simulink model "Quaternions_Method_merge_gio_giusto"  (R2021b)
settings: Solver=FixedStepAuto  StartTime=0.0  StopTime=Time  FixedStep=1  RelTol=1e-13  AbsTol=1e-8
values from neighbouring files (symbols this model uses):
  a = 8.6251e+06    (= 8625100)    [Main.m]
  c = 299792*10^3    (= 299792000)    [Main.m]
  e = 0.1195    [Main.m]
  G = 6.67259 * 1e-11    (= 6.67259e-11)    [Main.m]
  H_0 = sqrt((g_1_0)^2 + (g_1_1)^2 + (h_1_1)^2)    [Main.m]
  i = 0.3815    [Main.m]
  MB = [2000; 0.3; 1; 0.12].*1e-2    [Main.m]
  mr = 1.2 * 0.0001    (= 0.00012)    [Main.m]
  muP = G*Mt    (= 398527110340000)    [Main.m]
  omega_0 = [om_x, om_y, om_z]    [Main.m]
  p_acc = deg2rad(5)    [Main.m]
  RD = 0.1*ones(1,10)    [Main.m]
  RS_MB = 0.5    [Main.m]
  RS_SP = 0.1    [Main.m]
  SP = [2000; 0.3; 1; 0.12].*1e-2    [Main.m]
  theta0 = 0    [Main.m]
  w_E = (2*pi)/(24*3600)    (= 7.27220521664e-05)    [Main.m]
undefined symbols (not defined in the file or in its folder): A_BN_0, A_rw, A_rw_star, H, magnitude, rho_d_MB, rho_d_SP, rho_s_MB, rho_s_SP, sig_b, sig_n, T, t_sample
libraries: matrix_library x23, vrlib x9, simulink_extras x2, simulink x2
(part 8 of 8)

== system Quaternions_Method_merge_gio_giusto/Enviroment/Solar Radiation Perturbation/Sum forces/determine highlighted area/creazione della matrice che ha per colonne i vettori distanza tra il CM del MB e i centri geom delle aree illuminate dal sole /creazione raggi vettore tra CM MB e centro facce illuminate della faccia che ha come normale l'asse k/If Action Subsystem3 ==
  Action Port : ActionPort
  Constant : Constant  Value=[0;0;0]
  Out1 : Outport
  wires:
  Constant/1 -> Out1/1

== system Quaternions_Method_merge_gio_giusto/Enviroment/Solar Radiation Perturbation/Sum forces/determine highlighted area/creazione della matrice che ha per colonne i vettori distanza tra il CM del MB e i centri geom delle aree illuminate dal sole /creazione raggi vettore tra CM MB e centro facce illuminate della faccia che ha come normale l'asse k/If Action Subsystem4 ==
  Areas_vect : Inport
  MB1 : Inport  Port=2
  Action Port : ActionPort
  Add : Sum  Inputs=+|-
  Add1 : Sum  Inputs=+|-
  Add2 : Sum
  Demux : Demux  Outputs=3
  Demux1 : Demux  Outputs=3
  Demux2 : Demux
  Divide : Product  Inputs=*/
  Divide1 : Product  Inputs=*/
  Gain{,1..3} (4 alike) : Gain  Gain=1/2
  Gain4 : Gain  Gain=-1
  Ground : Ground
  Ground1 : Ground
  Mux : Mux  Inputs=3
  Mux1 : Mux  Inputs=3
  Reshape{,1..3} (4 alike) : Reshape  OutputDimensionality=Column vector (2-D)
  Terminator{,1..3,8..9} (6 alike) : Terminator
  r_cface_cluce_xneg_y_pos : Outport
  wires:
  Demux/2 -> Terminator8/1
  Demux/1 -> Terminator9/1
  Demux1/2 -> Terminator1/1
  Demux1/1 -> Terminator/1
  Add2/1 -> r_cface_cluce_xneg_y_pos/1
  Reshape3/1 -> Add2/2
  Reshape2/1 -> Add2/1
  Divide1/1 -> Gain3/1
  Reshape1/1 -> Demux1/1
  Gain2/1 -> Add1/1
  Gain3/1 -> Add1/2
  Demux1/3 -> Divide1/1
  Ground/1 -> Mux1/1, Mux1/3
  Mux1/1 -> Reshape3/1  "raggio vettore che collega il centro geom della faccia con il centro geom della faccia illuminata dal sole lungo j"
  Reshape/1 -> Demux/1
  Ground1/1 -> Mux/2, Mux/3
  Areas_vect/1 -> Reshape1/1, Reshape/1
  Gain/1 -> Add/1
  Demux/3 -> Divide/1
  Gain1/1 -> Add/2
  Mux/1 -> Reshape2/1  "raggio vettore che collega il centro geom della faccia con il centro geom della faccia illuminata dal sole lungo -i"
  Divide/1 -> Gain1/1
  [b_MB] -> Divide/2
  [a_MB] -> Gain/1
  Add/1 -> Gain4/1
  Gain4/1 -> Mux/1
  Add1/1 -> Mux1/2
  [b_MB] -> Gain2/1
  [a_MB] -> Divide1/2
  Demux2/1 -> Terminator2/1
  Demux2/2 -> [a_MB]
  MB1/1 -> Demux2/1
  Demux2/3 -> [b_MB]
  Demux2/4 -> Terminator3/1

== system Quaternions_Method_merge_gio_giusto/Enviroment/Solar Radiation Perturbation/Sum forces/determine highlighted area/creazione della matrice che ha per colonne i vettori distanza tra il CM del MB e i centri geom delle aree illuminate dal sole /creazione raggi vettore tra CM MB e centro facce illuminate della faccia che ha come normale l'asse k/If Action Subsystem5 ==
  Action Port : ActionPort
  Constant : Constant  Value=[0;0;0]
  Out1 : Outport
  wires:
  Constant/1 -> Out1/1

== system Quaternions_Method_merge_gio_giusto/Enviroment/Solar Radiation Perturbation/Sum forces/determine highlighted area/creazione della matrice che ha per colonne i vettori distanza tra il CM del MB e i centri geom delle aree illuminate dal sole /creazione raggi vettore tra CM MB e centro facce illuminate della faccia che ha come normale l'asse k/If Action Subsystem6 ==
  Action Port : ActionPort
  Constant : Constant  Value=[0;0;0]
  Out1 : Outport
  wires:
  Constant/1 -> Out1/1

== system Quaternions_Method_merge_gio_giusto/Enviroment/Solar Radiation Perturbation/Sum forces/determine highlighted area/creazione della matrice che ha per colonne i vettori distanza tra il CM del MB e i centri geom delle aree illuminate dal sole /creazione raggi vettore tra CM MB e centro facce illuminate della faccia che ha come normale l'asse k/If Action Subsystem7 ==
  Action Port : ActionPort
  Constant : Constant  Value=[0;0;0]
  Out1 : Outport
  wires:
  Constant/1 -> Out1/1

== system Quaternions_Method_merge_gio_giusto/Enviroment/Solar Radiation Perturbation/Sum forces/determine highlighted area/creazione della matrice che ha per colonne i vettori distanza tra il CM del MB e i centri geom delle aree illuminate dal sole /creazione raggi vettore tra CM MB e centro facce illuminate della faccia che ha come normale l'asse k/creating distance between cm MB and centro geom lato1 ==
  MB : Inport
  Demux : Demux
  Ground : Ground
  Mux : Mux  Inputs=3
  Reshape : Reshape  OutputDimensionality=Column vector (2-D)
  Terminator : Terminator
  Terminator2 : Terminator
  Terminator3 : Terminator
  Out1 : Outport
  wires:
  Reshape/1 -> Out1/1
  Mux/1 -> Reshape/1
  MB/1 -> Demux/1
  Demux/1 -> Terminator/1
  Demux/2 -> Mux/1
  Demux/3 -> Terminator2/1
  Ground/1 -> Mux/2, Mux/3
  Demux/4 -> Terminator3/1

== matlab function Quaternions_Method_merge_gio_giusto/Attitude determination/MATLAB Function ==
  data: K input; V output; D output
function [V, D] = fcn(K)
[V,D] = eig(K);
end

== matlab function Quaternions_Method_merge_gio_giusto/Enviroment/Magnetic torque /Magnetic field in body frame/MATLAB Function ==
  data: r_LVLH input; r input; b_N output; t input; G input; H input
function b_N  = magnet(r_LVLH, r, t, G, H)
% Inputs
% r Geocentric radius
% theta Latitude measured in degrees positive from equator
% phi Longitude measured in degrees positive east from Greenwich
%
% Outputs - magnetic field strength in local tangential coordinates
% Br B in radial direction
% Bt B in theta direction
% Bp B in phi direction

% Computing the right ascension alpha, the declination delta, the longitude lon and the co-latitude phi
r_norm = norm(r_LVLH);
delta = asin(r_LVLH(3)/r_norm);
if(r_LVLH(2)/r_norm > 0)
    alpha = acos((r_LVLH(1)/r_norm)/cos(delta));
else 
    alpha = 2*pi -  acos((r_LVLH(1)/r_norm)/cos(delta));
end
theta = -delta;
om_E = deg2rad(15.04)/3600;
Gren_lon = om_E*t;
phi = (alpha - Gren_lon);

% Checks to see if located at either pole to avoid singularities
if (theta>-0.00000001 && theta<0.00000001)
theta=0.00000001;
elseif(theta<180.00000001 && theta>179.99999999)
theta=179.99999999;
end
% The angles must be converted from degrees into radians
theta=(90-theta)*pi/180;
phi = phi*pi/180;
a=6371.2; % Reference radius used in IGRF
% This section of the code simply reads in the g and h Schmidt
% quasi-normalized coefficients
gn = G(:,1);
gm = G(:,2);
gvali = G(:,3);
hn = H(:,1);
hm = H(:,2);
hvali = H(:,3);
%[gn, gm, gvali, ~] = textread('igrfSg.txt','%f %f %f %f');
%[hn, hm, hvali, ~]= textread('igrfSh.txt','%f %f %f %f');
N=max(gn);
g=zeros(N,N+1);
h=zeros(N,N+1);
for x=1:length(gn)
g(gn(x),gm(x)+1) = gvali(x);
h(hn(x),hm(x)+1) = hvali(x);
end
% Initialize each of the variables
% Br B in the radial driection
% Bt B in the theta direction
% Bp B in the phi direction
% P The associated Legendre polynomial evaluated at cos(theta)
% The nomenclature for the recursive values generally follows
% the form P10 = P(n-1,m-0)
% dP The partial derivative of P with respect to theta
Br=0; Bt=0; Bp=0;
P11=1; P10=P11;
dP11=0; dP10=dP11;
for m=0:N
for n=1:N
if m<=n
% Calculate Legendre polynomials and derivatives recursively
if n==m
P2 = sin(theta)*P11;
dP2 = sin(theta)*dP11 + cos(theta)*P11;
P11=P2; P10=P11; P20=0;
dP11=dP2; dP10=dP11; dP20=0;
elseif n==1
P2 = cos(theta)*P10;
dP2 = cos(theta)*dP10 - sin(theta)*P10;
P20=P10; P10=P2;
dP20=dP10; dP10=dP2;
else
P20=P10;
dP20=dP10;
K = ((n-1)^2-m^2)/((2*n-1)*(2*n-3));
P2 = cos(theta)*P10 - K*P20;
dP2 = cos(theta)*dP10 - sin(theta)*P10 - K*dP20;
P10=P2;
dP10=dP2;
end
% Calculate Br, Bt, and Bp
Br = Br + (a/r)^(n+2)*(n+1)*...
((g(n,m+1)*cos(m*phi) + h(n,m+1)*sin(m*phi))*P2);
Bt = Bt + (a/r)^(n+2)*...
((g(n,m+1)*cos(m*phi) + h(n,m+1)*sin(m*phi))*dP2);
Bp = Bp + (a/r)^(n+2)*...
(m*(-g(n,m+1)*sin(m*phi) + h(n,m+1)*cos(m*phi))* P2);
end
end
end
% Spherical coordinates
Br = Br;
Bt = -Bt;
Bp = -Bp / sin(theta);

% Inertial cartesian coordinates
LST = Gren_lon + phi;
lat = theta;
Bx = (Br*cos(lat)+Bt*sin(lat))*cos(LST) - Bp*sin(LST);
By = (Br*cos(lat)+Bt*sin(lat))*sin(LST) + Bp*cos(LST);
Bz = (Br*sin(lat)+Bt*cos(lat));

b_N = [Bx; By; Bz];

end

== matlab function Quaternions_Method_merge_gio_giusto/Inertia matrix/MATLAB Function ==
  data: u input; V output; D output
function [V,D] = fcn(u)

[V,D] = eig(u);
end
